simulink model "FogRectificationHDL"  (R2024b)
settings: Solver=FixedStepDiscrete  StartTime=0.0  StopTime=2*T  RelTol=1e-3
InitFcn:
  | img_path = get_param('FogRectificationHDL/FogImage','FileName');
  | img = imread(img_path);
  | %[m,n,c] = size(img);
  | m = 240;
  | n = 320;
  | c = 3;
  | dimI = [m n 3];
  | g = m*n;
  | 
  | numPixels = prod(dimI);
  | h1 = [1, 2, 1; 2, 4, 2; 1, 2 ,1]./16 ;
  | h = fliplr(flipud(h1));
  | T =324*402; % total pixels per line*total video lines
  | 
  | numBins = 256;
  | hazeFactor = 0.9;
  | reductionFactor = 0.6;
  | normFactor =  1/g;
  | threshold1 = 0.05;
  | threshold2 = 0.95;
  | o1 = 25;
  | o2 = 229;
  | o2_1 = 204;
  | max_o2 = 26;
undefined symbols (not defined in the file or in its folder): gray, Rec, SDTV
libraries: simulink x40, hdlsllib x32, visionhdlutilities x2, visionhdlio x2, visionsources x1, visionhdlstatistics x1, visionhdlconversions x1, visionhdlfilter x1, visionzynq_privlib x1
(part 2 of 2)

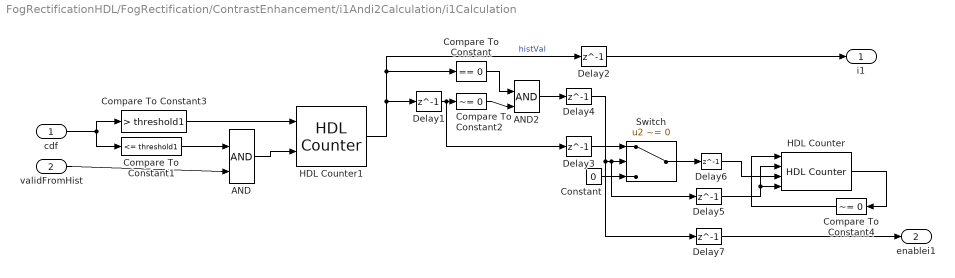
== system FogRectificationHDL/FogRectification/ContrastEnhancement/i1Andi2Calculation/i1Calculation   ==
  cdf : Inport
  validFromHist : Inport  Port=2
  AND : Logic  IconShape=distinctive  AllPortsSameDT=off  OutDataTypeStr=boolean
  AND2 : Logic  IconShape=distinctive  AllPortsSameDT=off  OutDataTypeStr=boolean
  Compare To Constant : simulink/Logic and Bit Operations/Compare To Constant  relop===  const=0  OutDataTypeStr=boolean
  Compare To Constant1 : simulink/Logic and Bit Operations/Compare To Constant  relop=<=  const=threshold1  OutDataTypeStr=boolean
  Compare To Constant2 : simulink/Logic and Bit Operations/Compare To Constant  relop=~=  const=0  OutDataTypeStr=boolean
  Compare To Constant3 : simulink/Logic and Bit Operations/Compare To Constant  relop=>  const=threshold1  OutDataTypeStr=boolean
  Compare To Constant4 : simulink/Logic and Bit Operations/Compare To Constant  relop=~=  const=0  OutDataTypeStr=boolean
  Constant : Constant  Value=0  OutDataTypeStr=uint8  SampleTime=-1
  Delay{1..7} (7 alike) : Delay  DelayLength=1
  HDL Counter : hdlsllib/Sources/HDL Counter  CountType=Count limited  CountInit=0  CountStep=1  CountMax=25  CountFromType=Initial value  CountFrom=0  CountResetPort=on  CountLoadPort=on  CountEnbPort=on  CountDirPort=off  CountHitOutputPort=off  CountDataType=Unsigned  CountWordLen=8  CountFracLen=0  CountSampTime=1
  HDL Counter1 : hdlsllib/Sources/HDL Counter  CountType=Free running  CountInit=0  CountStep=1  CountMax=255  CountFromType=Initial value  CountFrom=0  CountResetPort=on  CountLoadPort=off  CountEnbPort=on  CountDirPort=off  CountHitOutputPort=off  CountDataType=Unsigned  CountWordLen=ceil(log2(numBins))  CountFracLen=0  CountSampTime=1
  Switch : Switch  Criteria=u2 ~= 0  SaturateOnIntegerOverflow=off  InputSameDT=off
  i1 : Outport
  enablei1 : Outport  Port=2
  wires:
  HDL Counter/1 -> Compare To Constant4/1
  Delay1/1 -> Delay3/1, Compare To Constant2/1
  Constant/1 -> Switch/3
  validFromHist/1 -> AND/2
  Compare To Constant1/1 -> AND/1
  cdf/1 -> Compare To Constant3/1, Compare To Constant1/1
  AND2/1 -> Delay4/1
  HDL Counter1/1 -> Compare To Constant/1, Delay2/1, Delay1/1  "histVal"
  Compare To Constant3/1 -> HDL Counter1/1
  Compare To Constant2/1 -> AND2/2
  Compare To Constant/1 -> AND2/1
  AND/1 -> HDL Counter1/2
  Delay2/1 -> i1/1
  Delay3/1 -> Switch/1
  Delay4/1 -> Delay5/1, Switch/2, Delay7/1
  Delay5/1 -> HDL Counter/2, HDL Counter/4
  Switch/1 -> Delay6/1
  Delay6/1 -> HDL Counter/3
  Compare To Constant4/1 -> HDL Counter/1
  Delay7/1 -> enablei1/1

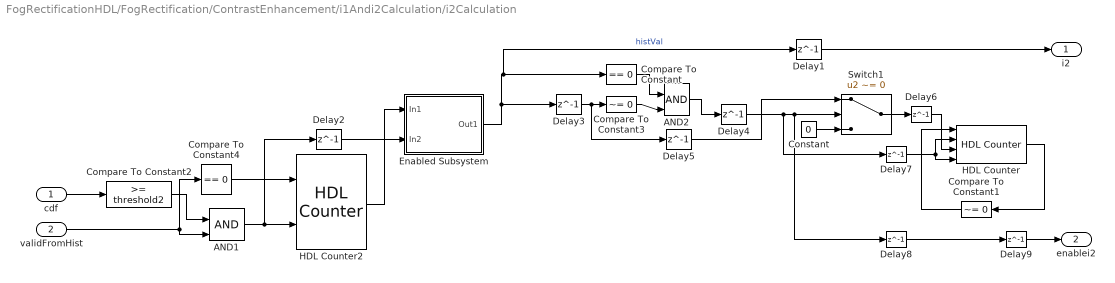
== system FogRectificationHDL/FogRectification/ContrastEnhancement/i1Andi2Calculation/i2Calculation ==
  cdf : Inport
  validFromHist : Inport  Port=2
  AND1 : Logic  IconShape=distinctive  AllPortsSameDT=off  OutDataTypeStr=boolean
  AND2 : Logic  IconShape=distinctive  AllPortsSameDT=off  OutDataTypeStr=boolean
  Compare To Constant : simulink/Logic and Bit Operations/Compare To Constant  relop===  const=0  OutDataTypeStr=boolean
  Compare To Constant1 : simulink/Logic and Bit Operations/Compare To Constant  relop=~=  const=0  OutDataTypeStr=boolean
  Compare To Constant2 : simulink/Logic and Bit Operations/Compare To Constant  relop=>=  const=threshold2  OutDataTypeStr=boolean
  Compare To Constant3 : simulink/Logic and Bit Operations/Compare To Constant  relop=~=  const=0  OutDataTypeStr=boolean
  Compare To Constant4 : simulink/Logic and Bit Operations/Compare To Constant  relop===  const=0  OutDataTypeStr=boolean
  Constant : Constant  Value=0  OutDataTypeStr=uint8  SampleTime=-1
  Delay{1..9} (9 alike) : Delay  DelayLength=1
  Enabled Subsystem : Subsystem  TreatAsAtomicUnit=on
  HDL Counter : hdlsllib/Sources/HDL Counter  CountType=Count limited  CountInit=0  CountStep=1  CountMax=25  CountFromType=Initial value  CountFrom=0  CountResetPort=on  CountLoadPort=on  CountEnbPort=on  CountDirPort=off  CountHitOutputPort=off  CountDataType=Unsigned  CountWordLen=8  CountFracLen=0  CountSampTime=1
  HDL Counter2 : hdlsllib/Sources/HDL Counter  CountType=Free running  CountInit=0  CountStep=1  CountMax=255  CountFromType=Initial value  CountFrom=0  CountResetPort=on  CountLoadPort=off  CountEnbPort=on  CountDirPort=off  CountHitOutputPort=off  CountDataType=Unsigned  CountWordLen=ceil(log2(numBins))  CountFracLen=0  CountSampTime=1
  Switch1 : Switch  Criteria=u2 ~= 0  SaturateOnIntegerOverflow=off  InputSameDT=off
  i2 : Outport
  enablei2 : Outport  Port=2
  wires:
  AND1/1 -> Delay2/1, HDL Counter2/2
  Compare To Constant2/1 -> AND1/1
  HDL Counter2/1 -> Enabled Subsystem/1(In1)
  cdf/1 -> Compare To Constant2/1
  validFromHist/1 -> Compare To Constant4/1, AND1/2
  Compare To Constant4/1 -> HDL Counter2/1
  Delay2/1 -> Enabled Subsystem/2(In2)
  Compare To Constant3/1 -> AND2/2
  Compare To Constant/1 -> AND2/1
  Enabled Subsystem/1(Out1) -> Delay3/1, Delay1/1, Compare To Constant/1  "histVal"
  AND2/1 -> Delay4/1
  Constant/1 -> Switch1/3
  HDL Counter/1 -> Compare To Constant1/1
  Switch1/1 -> Delay6/1
  Delay3/1 -> Delay5/1, Compare To Constant3/1
  Delay1/1 -> i2/1
  Delay4/1 -> Delay8/1, Switch1/2, Delay7/1
  Delay5/1 -> Switch1/1
  Delay6/1 -> HDL Counter/3
  Delay7/1 -> HDL Counter/2, HDL Counter/4
  Delay8/1 -> Delay9/1
  Compare To Constant1/1 -> HDL Counter/1
  Delay9/1 -> enablei2/1

== system FogRectificationHDL/FogRectification/FogRemoval/Restoration/DiffOfInputAndDiffim ==
  diffimAfterReduction : Inport
  ScaledInput : Inport  Port=2
  ctrlIn : Inport  Port=3
  Constant1 : Constant  Value=reductionFactor  OutDataTypeStr=fixdt(0,16,15)  SampleTime=-1
  Delay{,1..6} (7 alike) : Delay
  Delay{7..10} (4 alike) : Delay  DelayLength=1
  Product : Product  OutDataTypeStr=fixdt(0,32,20)
  Subtract : Sum  Inputs=+-
  diffOfIpAnddiffim : Outport
  diffimForRst : Outport  Port=2
  ctrlOut : Outport  Port=3
  wires:
  Subtract/1 -> Delay7/1
  Delay/1 -> Delay8/1, Subtract/2
  Delay2/1 -> Delay9/1
  ctrlIn/1 -> Delay5/1
  ScaledInput/1 -> Delay6/1
  diffimAfterReduction/1 -> Delay3/1
  Product/1 -> Delay10/1
  Delay1/1 -> Subtract/1
  Constant1/1 -> Delay4/1
  Delay3/1 -> Product/1
  Delay4/1 -> Product/2
  Delay5/1 -> Delay2/1
  Delay7/1 -> diffOfIpAnddiffim/1
  Delay8/1 -> diffimForRst/1
  Delay9/1 -> ctrlOut/1
  Delay6/1 -> Delay1/1
  Delay10/1 -> Delay/1

== system FogRectificationHDL/FogRectification/FogRemoval/Restoration/FactorCalculation ==
  diffimForRestoration : Inport
  Constant1 : Constant  Value=255  OutDataTypeStr=uint8  SampleTime=-1
  Constant2 : Constant  Value=255  OutDataTypeStr=uint8  SampleTime=-1
  Delay{1,3,12,15} (4 alike) : Delay
  Delay10 : Delay  DelayLength=1
  Delay14 : Delay  DelayLength=44
  Delay2 : Delay  DelayLength=44
  Delay9 : Delay  DelayLength=1
  Product : Product  Inputs=/  RndMeth=Zero  SaturateOnIntegerOverflow=on
  Product2 : Product
  Subtract1 : Sum  Inputs=+-  OutDataTypeStr=fixdt(0,40,25)  RndMeth=Nearest
  factor : Outport
  wires:
  Subtract1/1 -> Delay15/1
  diffimForRestoration/1 -> Delay10/1
  Constant2/1 -> Delay9/1
  Delay10/1 -> Subtract1/2
  Delay9/1 -> Subtract1/1
  Product2/1 -> Delay12/1
  Delay12/1 -> factor/1
  Delay14/1 -> Delay3/1
  Product/1 -> Delay14/1
  Delay15/1 -> Product/1
  Constant1/1 -> Delay2/1
  Delay2/1 -> Delay1/1
  Delay1/1 -> Product2/1
  Delay3/1 -> Product2/2

== system FogRectificationHDL/ImageBuffer/BehavioralMemory/BehavioralMemory/pixelBusGenerator ==
  validIn : Inport
  Horizontal : hdlsllib/Sources/HDL Counter  CountType=Count limited  CountInit=0  CountStep=1  CountMax=hEnd  CountFromType=Initial value  CountFrom=0  CountResetPort=off  CountLoadPort=off  CountEnbPort=on  CountDirPort=off  CountHitOutputPort=off  CountDataType=Unsigned  CountWordLen=ceil(log2(hEnd))  CountFracLen=0  CountSampTime=1
  Logical Operator{3..6} (4 alike) : Logic  AllPortsSameDT=off  OutDataTypeStr=boolean
  Pixel Control Bus Creator : visionhdlutilities/Pixel Control Bus Creator
  Vertical : hdlsllib/Sources/HDL Counter  CountType=Count limited  CountInit=0  CountStep=1  CountMax=vEnd  CountFromType=Initial value  CountFrom=0  CountResetPort=off  CountLoadPort=off  CountEnbPort=on  CountDirPort=off  CountHitOutputPort=off  CountDataType=Unsigned  CountWordLen=ceil(log2(vEnd))  CountFracLen=0  CountSampTime=1
  hEnd : simulink/Logic and Bit Operations/Compare To Constant  relop===  const=hEnd  OutDataTypeStr=boolean
  hStart : simulink/Logic and Bit Operations/Compare To Constant  relop===  const=0  OutDataTypeStr=boolean
  vEnd : simulink/Logic and Bit Operations/Compare To Constant  relop===  const=vEnd  OutDataTypeStr=boolean
  vStart : simulink/Logic and Bit Operations/Compare To Constant  relop===  const=0  OutDataTypeStr=boolean
  busOut : Outport  VectorParamsAs1DForOutWhenUnconnected=off
  wires:
  validIn/1 -> Pixel Control Bus Creator/5, Vertical/1, Logical Operator4/1, Logical Operator5/1, Logical Operator6/1, Logical Operator3/1, Horizontal/1
  Horizontal/1 -> hEnd/1, hStart/1
  hEnd/1 -> Logical Operator4/2
  Vertical/1 -> vStart/1, vEnd/1
  vStart/1 -> Logical Operator5/2
  vEnd/1 -> Logical Operator6/2
  Logical Operator5/1 -> Pixel Control Bus Creator/3
  Logical Operator3/1 -> Pixel Control Bus Creator/1
  Logical Operator4/1 -> Pixel Control Bus Creator/2
  hStart/1 -> Logical Operator3/2
  Logical Operator6/1 -> Pixel Control Bus Creator/4
  Pixel Control Bus Creator/1 -> busOut/1

== system FogRectificationHDL/FogRectification/ContrastEnhancement/i1Andi2Calculation/i2Calculation/Enabled Subsystem ==
  In1 : Inport
  In2 : Inport  Port=2
  Constant : Constant  Value=255  OutDataTypeStr=uint8  SampleTime=-1
  Constant1 : Constant  Value=0  OutDataTypeStr=uint8  SampleTime=-1
  Delay : Delay  DelayLength=1
  Delay1 : Delay  DelayLength=1
  Subtract : Sum  Inputs=+-  OutDataTypeStr=uint8
  Switch : Switch  Criteria=u2 ~= 0  SaturateOnIntegerOverflow=off  InputSameDT=off
  Out1 : Outport  InitialOutput=0  VectorParamsAs1DForOutWhenUnconnected=off
  wires:
  Constant/1 -> Subtract/1
  In1/1 -> Subtract/2  "histVal1"
  Subtract/1 -> Delay/1
  In2/1 -> Delay1/1  "histVal1"
  Switch/1 -> Out1/1
  Constant1/1 -> Switch/3
  Delay/1 -> Switch/1
  Delay1/1 -> Switch/2
